simulink model "gm_sampleModel1485_3_sub"  (R2023a)
settings: Solver=VariableStepAuto  StartTime=0.0  StopTime=10.0  RelTol=1e-3
libraries: simulink x2, hdlsllib x1
settings Model: Creator=user1  LastModifiedBy=user1
settings OptimizationCC: BlockReduction=off  ConditionallyExecuteInputs=off
settings DebuggingCC: InheritedTsInSrcMsg=none

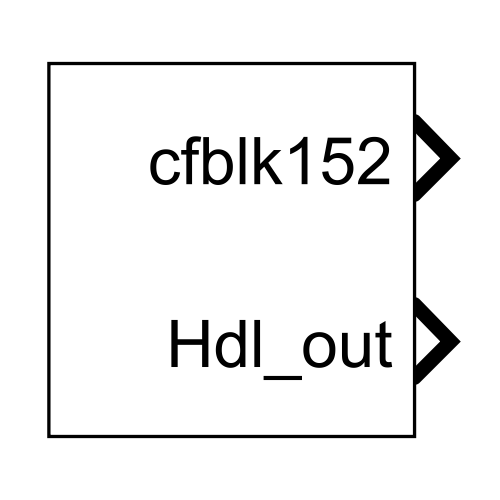
[thumbnail: Simulink's stored preview of the top-level diagram]
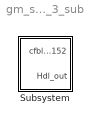
== system gm_sampleModel1485_3_sub ==
  Subsystem : Subsystem

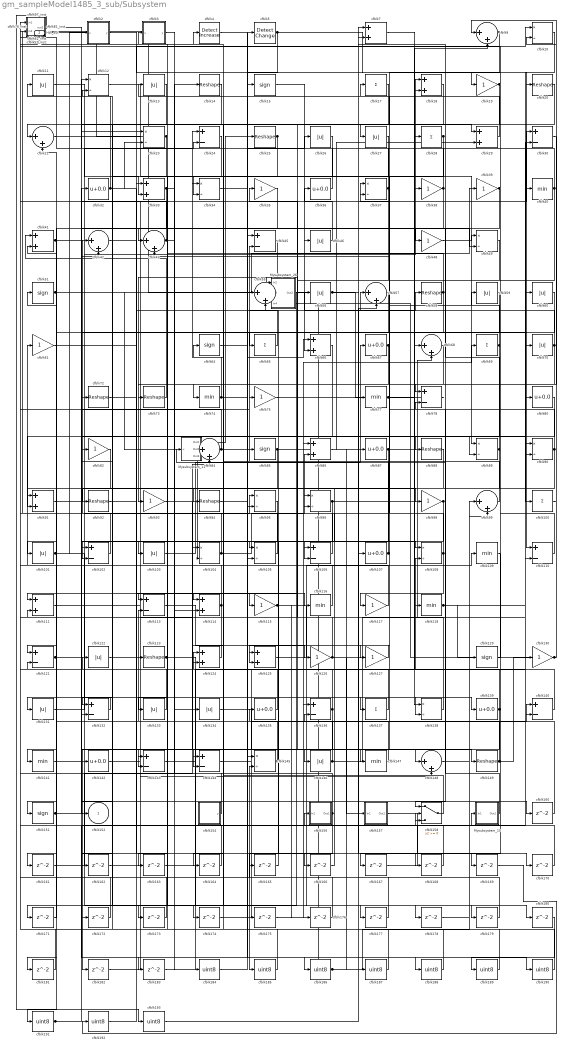
== system gm_sampleModel1485_3_sub/Subsystem ==
  Mysubsystem_10 : Subsystem
  Mysubsystem_11 : Subsystem
  Mysubsystem_26 : Subsystem
  cfblk{10,12,23,34,37,49,89..90,95..96,104..105,108,138,145} (15 alike) : Product  Inputs=*/  OutDataTypeStr=uint8  RndMeth=Zero  SaturateOnIntegerOverflow=on
  cfblk{17,28,65,69,100,137} (6 alike) : Sum  Inputs=+  OutDataTypeStr=uint8
  cfblk{11,13,26..27,46,56,59..60,70,101,103,122,131,133..134,146} (16 alike) : Abs  OutDataTypeStr=uint8  SaturateOnIntegerOverflow=off
  cfblk{24,30,45,78,102,106,110,113,121,132,136,140,143..144} (14 alike) : Sum  Inputs=+-  OutDataTypeStr=uint8
  cfblk{32,36,67,80,87,107,135,139,142} (9 alike) : Bias  Bias=0.0  SaturateOnIntegerOverflow=off
  cfblk{40,74,77,109,116,118,141,147} (8 alike) : MinMax  OutDataTypeStr=uint8
  cfblk{7,18,29,33,41,66,86,91,111,114,124..125} (12 alike) : Sum  OutDataTypeStr=uint8
  cfblk{19,35,38..39,48,61,75,82,93,98,115,117,126..127,130} (15 alike) : Gain  OutDataTypeStr=uint8
  cfblk{14,20,25,58,72..73,88,92,94,123,149} (11 alike) : Reshape
  cfblk{15,51,64,85,129,151} (6 alike) : Signum
  cfblk{9,21,42..43,55,57,68,84,99,148} (10 alike) : Sum  Inputs=|++  OutDataTypeStr=uint8
  cfblk150_inst : Subsystem
  cfblk154 : Subsystem  mask(Counter Free-Running){NumBits=double(16), tsamp=double(-1)}
      mask prompts: NumBits "Simulink:masks:NumberOfBits_MP"; tsamp "Simulink:masks:SampleTime_MP"
      mask help: Simulink:masks:CounterFreeRunning_MD
  cfblk156 : Subsystem
  cfblk157 : Subsystem
  cfblk158 : Switch  OutDataTypeStr=uint8  SaturateOnIntegerOverflow=off  InputSameDT=off
  cfblk{160..183} (24 alike) : Delay  SampleTime=1
  cfblk16_inst : Subsystem
  cfblk{184..193} (10 alike) : DataTypeConversion  OutDataTypeStr=uint8  SaturateOnIntegerOverflow=off  RndMeth=Floor
  cfblk2 : Subsystem  mask(Compare To Zero){relop=<=, OutDataTypeStr=uint8, ZeroCross=on}
      mask prompts: relop "Simulink:masks:Operator_MP"; OutDataTypeStr "Simulink:masks:OutputDataType_MP"; ZeroCross "Simulink:masks:EnableZerocrossingDetection_MP"
      mask help: Simulink:masks:CompareToZero_MD
      mask init:
      | OutDataTypeStr = 'uint8';
      | ZeroCross = 'on';
      | blkName = 'sampleModel1485_3_sub/Subsystem/cfblk2';
      | relop = '<=';
      | setValue = 'fixdt(0, 8)';
      mask TypeOptions relop: == | ~= | < | <= | >= | >
      mask TypeOptions OutDataTypeStr: Simulink:masks:uint8 | Simulink:masks:boolean
      mask Callback ZeroCross: sl('zeroCrossEnable', gcbh);
      mask Display: disp([relop,' 0'])
  cfblk22_inst : Subsystem
  cfblk3 : Subsystem  mask(Compare To Constant){relop=<=, const=double(3), OutDataTypeStr=uint8, ZeroCross=on}
      mask prompts: relop "Simulink:masks:Operator_MP"; const "Simulink:masks:ConstantValue_MP"; OutDataTypeStr "Simulink:masks:OutputDataType_MP"; ZeroCross "Simulink:masks:EnableZerocrossingDetection_MP"
      mask help: Simulink:masks:CompareToConstant_MD
      mask init:
      | OutDataTypeStr = 'uint8';
      | ZeroCross = 'on';
      | blkName = 'sampleModel1485_3_sub/Subsystem/cfblk3';
      | const = double(3);
      | const_str = '3.0';
      | const_val = double(3);
      | relop = '<=';
      | setValue = 'fixdt(0, 8)';
      | str = '<= 3';
      mask TypeOptions relop: == | ~= | < | <= | >= | >
      mask TypeOptions OutDataTypeStr: Simulink:masks:uint8 | Simulink:masks:boolean
      mask Callback ZeroCross: sl('zeroCrossEnable', gcbh);
      mask Display: disp(str)
  cfblk31_inst : Subsystem
  cfblk4 : simulink/Logic and Bit Operations/Detect Increase  vinit=0.0  OutDataTypeStr=uint8
      settings: LibrarySourceBlock=|
      | hdlsllib/Logic and Bit
      | Operations/Detect
      | Increase
  cfblk47_inst : Subsystem
  cfblk5 : simulink/Logic and Bit Operations/Detect Change  vinit=0  OutDataTypeStr=uint8
      settings: LibrarySourceBlock=|
      | hdlsllib/Logic and Bit
      | Operations/Detect
      | Change
  cfblk52_inst : Subsystem
  cfblk54_inst : Subsystem
  cfblk62_inst : Subsystem
  cfblk76_inst : Subsystem
  cfblk81_inst : Subsystem
  cfblk97_inst : Subsystem
  cfblk152 : Outport  OutDataTypeStr=uint8  SampleTime=1  VectorParamsAs1DForOutWhenUnconnected=off
  Hdl_out : Outport  Port=2  OutDataTypeStr=uint8  SampleTime=1
  wires:
  Mysubsystem_10/1(Out1) -> Mysubsystem_11/1(u)
  Mysubsystem_11/1(Out1) -> cfblk25/1
  Mysubsystem_11/2(Out2) -> cfblk29/2
  Mysubsystem_11/3(Out3) -> cfblk104/2
  Mysubsystem_26/1(Out2) -> cfblk171/1
  cfblk10/1 -> cfblk110/1
  cfblk100/1 -> cfblk9/1
  cfblk101/1 -> cfblk24/2, cfblk95/1, cfblk178/1, cfblk2/1(u)
  cfblk102/1 -> cfblk42/1
  cfblk103/1 -> cfblk67/1
  cfblk104/1 -> cfblk86/2, cfblk54_inst/2(in2)
  cfblk105/1 -> cfblk97_inst/1(in1)
  cfblk106/1 -> cfblk96/1
  cfblk107/1 -> cfblk45/2, cfblk150_inst/1(in1)
  cfblk108/1 -> cfblk45/1, cfblk117/1, cfblk17/1
  cfblk109/1 -> cfblk167/1
  cfblk11/1 -> cfblk33/2
  cfblk110/1 -> cfblk81_inst/2(in2)
  cfblk111/1 -> cfblk58/1
  cfblk113/1 -> cfblk125/2
  cfblk114/1 -> cfblk22_inst/1(in1), cfblk111/2
  cfblk115/1 -> cfblk177/1, cfblk176/1
  cfblk116/1 -> cfblk35/1
  cfblk117/1 -> cfblk61/1
  cfblk118/1 -> cfblk60/1, cfblk129/1
  cfblk12/1 -> cfblk89/1
  cfblk121/1 -> cfblk18/1, cfblk139/1, cfblk181/1
  cfblk122/1 -> cfblk5/1
  cfblk123/1 -> cfblk180/1, cfblk179/1
  cfblk124/1 -> cfblk16_inst/1(in1)
  cfblk125/1 -> cfblk109/1
  cfblk126/1 -> cfblk68/2, cfblk157/1(In1), Mysubsystem_26/1(In2)
  cfblk127/1 -> cfblk125/1
  cfblk129/1 -> cfblk59/1
  cfblk13/1 -> cfblk21/1
  cfblk130/1 -> cfblk10/2, Mysubsystem_26/3(In4)
  cfblk131/1 -> cfblk15/1
  cfblk132/1 -> cfblk131/1
  cfblk133/1 -> cfblk122/1
  cfblk134/1 -> cfblk149/1
  cfblk135/1 -> cfblk72/1
  cfblk136/1 -> cfblk85/1, cfblk182/1
  cfblk137/1 -> cfblk124/1
  cfblk138/1 -> cfblk97_inst/2(in2)
  cfblk139/1 -> cfblk142/1, cfblk108/2
  cfblk14/1 -> cfblk102/2
  cfblk140/1 -> cfblk47_inst/1(in1)
  cfblk141/1 -> cfblk75/1
  cfblk142/1 -> cfblk30/1
  cfblk143/1 -> cfblk18/2
  cfblk144/1 -> cfblk68/1
  cfblk145/1 -> cfblk51/1, cfblk135/1
  cfblk146/1 -> cfblk30/2, cfblk113/2
  cfblk147/1 -> cfblk136/2
  cfblk148/1 -> cfblk140/1
  cfblk149/1 -> cfblk78/2, cfblk130/1
  cfblk15/1 -> cfblk66/2
  cfblk150_inst/1(out1) -> cfblk193/1
  cfblk151/1 -> cfblk32/1, cfblk14/1
  cfblk154/1(y) -> cfblk121/2
  cfblk156/1(Out1) -> cfblk31_inst/1(in1), cfblk185/1
  cfblk157/1(Out1) -> cfblk170/1
  cfblk158/1 -> cfblk64/1
  cfblk16_inst/1(out1) -> cfblk42/2
  cfblk160/1 -> cfblk86/1
  cfblk161/1 -> cfblk104/1
  cfblk162/1 -> cfblk148/2
  cfblk163/1 -> cfblk158/2
  cfblk164/1 -> cfblk81_inst/1(in1)
  cfblk165/1 -> cfblk55/2
  cfblk166/1 -> cfblk96/2
  cfblk167/1 -> cfblk90/1
  cfblk168/1 -> cfblk33/1
  cfblk169/1 -> cfblk192/1
  cfblk17/1 -> cfblk102/1
  cfblk170/1 -> cfblk136/1
  cfblk171/1 -> cfblk21/2
  cfblk172/1 -> cfblk52_inst/1(in1)
  cfblk173/1 -> cfblk150_inst/2(in2)
  cfblk174/1 -> cfblk99/2
  cfblk175/1 -> cfblk158/3
  cfblk176/1 -> cfblk145/2
  cfblk177/1 -> cfblk12/2
  cfblk178/1 -> cfblk140/2
  cfblk179/1 -> cfblk41/2
  cfblk18/1 -> cfblk124/2
  cfblk180/1 -> cfblk189/1
  cfblk181/1 -> cfblk62_inst/2(in2)
  cfblk182/1 -> cfblk84/2
  cfblk183/1 -> cfblk110/2
  cfblk184/1 -> cfblk26/1
  cfblk185/1 -> cfblk3/1(u)
  cfblk186/1 -> cfblk99/1, cfblk87/1
  cfblk187/1 -> cfblk4/1
  cfblk188/1 -> cfblk82/1
  cfblk189/1 -> cfblk76_inst/1(in1)
  cfblk19/1 -> cfblk34/2, cfblk174/1
  cfblk190/1 -> cfblk76_inst/2(in2)
  cfblk191/1 -> cfblk156/1(In1), Mysubsystem_10/1(In1)
  cfblk192/1 -> cfblk57/1
  cfblk193/1 -> cfblk57/2
  cfblk2/1(y) -> cfblk20/1
  cfblk20/1 -> cfblk115/1
  cfblk21/1 -> cfblk118/1
  cfblk22_inst/1(out1) -> cfblk29/1
  cfblk23/1 -> Hdl_out/1, cfblk152/1
  cfblk24/1 -> cfblk172/1
  cfblk25/1 -> cfblk94/1, cfblk43/1
  cfblk26/1 -> cfblk46/1
  cfblk27/1 -> cfblk92/1
  cfblk28/1 -> cfblk173/1, cfblk127/1
  cfblk29/1 -> cfblk13/1
  cfblk3/1(y) -> cfblk184/1
  cfblk30/1 -> cfblk80/1
  cfblk31_inst/1(out1) -> cfblk65/1
  cfblk32/1 -> cfblk144/2, cfblk11/1, cfblk23/2
  cfblk33/1 -> cfblk91/2, cfblk134/1
  cfblk34/1 -> cfblk70/1
  cfblk35/1 -> cfblk161/1
  cfblk36/1 -> cfblk31_inst/2(in2)
  cfblk37/1 -> cfblk54_inst/1(in1), cfblk111/1
  cfblk38/1 -> cfblk28/1, cfblk74/1
  cfblk39/1 -> cfblk78/1, cfblk48/1
  cfblk4/1 -> cfblk186/1
  cfblk40/1 -> cfblk143/2, cfblk12/1
  cfblk41/1 -> cfblk151/1, cfblk37/1, cfblk160/1
  cfblk42/1 -> cfblk116/1
  cfblk43/1 -> cfblk22_inst/2(in2), cfblk114/2
  cfblk45/1 -> cfblk93/1
  cfblk46/1 -> cfblk36/1
  cfblk47_inst/1(out1) -> cfblk90/2
  cfblk48/1 -> cfblk49/1
  cfblk49/1 -> cfblk73/1
  cfblk5/1 -> cfblk175/1, cfblk100/1
  cfblk51/1 -> cfblk84/1, cfblk39/1
  cfblk52_inst/1(out1) -> cfblk190/1, cfblk23/1
  cfblk54_inst/1(out1) -> cfblk105/1, cfblk137/1
  cfblk55/1 -> cfblk47_inst/2(in2), cfblk187/1
  cfblk56/1 -> cfblk7/2, cfblk169/1
  cfblk57/1 -> cfblk191/1
  cfblk58/1 -> cfblk16_inst/2(in2), cfblk121/1
  cfblk59/1 -> cfblk148/1
  cfblk60/1 -> cfblk105/2
  cfblk61/1 -> cfblk123/1
  cfblk62_inst/1(out1) -> cfblk49/2
  cfblk64/1 -> cfblk145/1
  cfblk65/1 -> cfblk55/1
  cfblk66/1 -> cfblk91/1
  cfblk67/1 -> cfblk95/2, cfblk147/1
  cfblk68/1 -> cfblk164/1
  cfblk69/1 -> cfblk43/2, cfblk114/1
  cfblk7/1 -> cfblk38/1
  cfblk70/1 -> cfblk88/1, cfblk56/1
  cfblk72/1 -> cfblk10/1
  cfblk73/1 -> cfblk41/1
  cfblk74/1 -> cfblk24/1, cfblk126/1
  cfblk75/1 -> cfblk77/1
  cfblk76_inst/1(out1) -> cfblk188/1
  cfblk77/1 -> cfblk89/2, cfblk40/1
  cfblk78/1 -> Mysubsystem_26/2(In3)
  cfblk80/1 -> cfblk101/1
  cfblk81_inst/1(out1) -> cfblk103/1, cfblk183/1
  cfblk82/1 -> cfblk141/1
  cfblk84/1 -> cfblk62_inst/1(in1), cfblk138/2
  cfblk85/1 -> cfblk132/1, cfblk69/1
  cfblk86/1 -> cfblk107/1
  cfblk87/1 -> cfblk9/2, cfblk106/2
  cfblk88/1 -> cfblk113/1
  cfblk89/1 -> cfblk7/1, cfblk158/1, cfblk132/2
  cfblk9/1 -> cfblk27/1, cfblk19/1
  cfblk90/1 -> cfblk106/1, cfblk37/2
  cfblk91/1 -> cfblk34/1
  cfblk92/1 -> cfblk168/1
  cfblk93/1 -> cfblk146/1
  cfblk94/1 -> cfblk66/1
  cfblk95/1 -> cfblk133/1
  cfblk96/1 -> cfblk162/1, cfblk138/1
  cfblk97_inst/1(out1) -> cfblk143/1, cfblk98/1, cfblk166/1, cfblk108/1
  cfblk98/1 -> cfblk144/1, cfblk165/1, cfblk163/1
  cfblk99/1 -> cfblk52_inst/2(in2)

== system gm_sampleModel1485_3_sub/Subsystem/Mysubsystem_10 ==
  In1 : Inport  OutDataTypeStr=uint8  PortDimensions=1  SampleTime=1
  cfblk159 : Delay  SampleTime=1
  Out1 : Outport  SampleTime=1
  wires:
  In1/1 -> cfblk159/1
  cfblk159/1 -> Out1/1

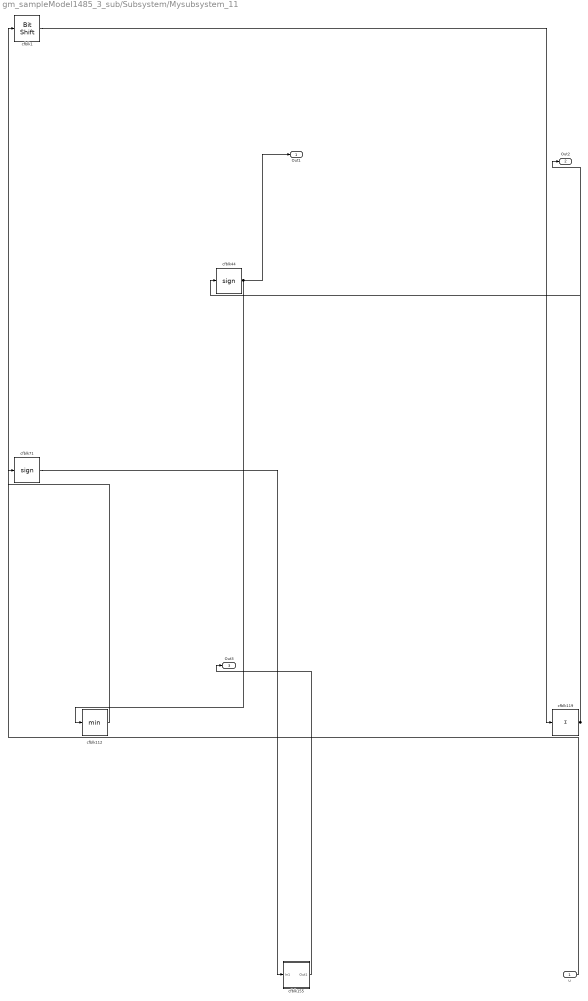
== system gm_sampleModel1485_3_sub/Subsystem/Mysubsystem_11 ==
  u : Inport  OutDataTypeStr=uint8  PortDimensions=1  SampleTime=1
  cfblk1 : hdlsllib/Logic and Bit Operations/Bit Shift  mode=Shift Left Logical  N=0
  cfblk112 : MinMax
  cfblk119 : Sum  Inputs=+
  cfblk155 : Subsystem
  cfblk44 : Signum
  cfblk71 : Signum
  Out1 : Outport  SampleTime=1
  Out2 : Outport  Port=2  SampleTime=1
  Out3 : Outport  Port=3  SampleTime=1
  wires:
  u/1 -> cfblk1/1
  cfblk1/1 -> cfblk119/1
  cfblk112/1 -> cfblk71/1
  cfblk119/1 -> cfblk44/1, Out2/1
  cfblk155/1(Out1) -> Out3/1
  cfblk44/1 -> Out1/1, cfblk112/1
  cfblk71/1 -> cfblk155/1(In1)

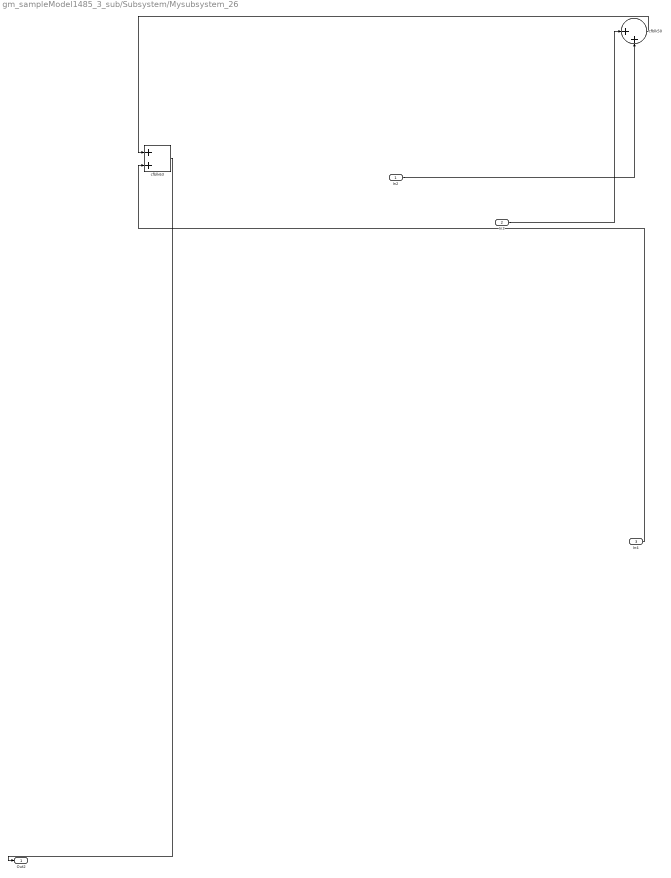
== system gm_sampleModel1485_3_sub/Subsystem/Mysubsystem_26 ==
  In2 : Inport  OutDataTypeStr=uint8  PortDimensions=1  SampleTime=1
  In3 : Inport  Port=2  OutDataTypeStr=uint8  PortDimensions=1  SampleTime=1
  In4 : Inport  Port=3  OutDataTypeStr=uint8  PortDimensions=1  SampleTime=1
  cfblk50 : Sum  Inputs=|++
  cfblk63 : Sum
  Out2 : Outport  SampleTime=1
  wires:
  In2/1 -> cfblk50/2
  In3/1 -> cfblk50/1
  In4/1 -> cfblk63/2
  cfblk50/1 -> cfblk63/1
  cfblk63/1 -> Out2/1

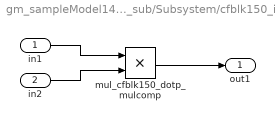
== system gm_sampleModel1485_3_sub/Subsystem/cfblk150_inst ==
  in1 : Inport  OutDataTypeStr=uint8  SampleTime=1
  in2 : Inport  Port=2  OutDataTypeStr=uint8  SampleTime=1
  mul_cfblk150_dotp_mulcomp : Product  Inputs=**  OutDataTypeStr=uint8  SampleTime=1
  out1 : Outport  OutDataTypeStr=uint8  SampleTime=1
  wires:
  in1/1 -> mul_cfblk150_dotp_mulcomp/1
  in2/1 -> mul_cfblk150_dotp_mulcomp/2
  mul_cfblk150_dotp_mulcomp/1 -> out1/1

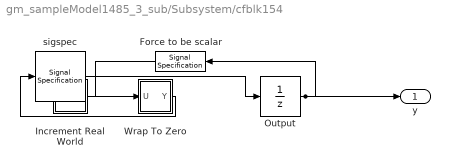
== system gm_sampleModel1485_3_sub/Subsystem/cfblk154 ==
  Force to be scalar : SignalSpecification  DisableCoverage=on  Dimensions=1
  Increment Real World : Subsystem  mask(Real World Value Increment){}
      mask help: Simulink:masks:RealWorldValueIncrement_MD
      mask Display: disp('V++')
  Output : UnitDelay  InitialCondition=0.0  SampleTime=tsamp  HasFrameUpgradeWarning=on
  Wrap To Zero : Subsystem  mask(Wrap To Zero){Threshold=double(65535)}
      mask prompts: Threshold "Simulink:masks:Threshold_MP"
      mask help: Simulink:masks:WrapToZero_MD
  sigspec : SignalSpecification  OutDataTypeStr=uint16  Dimensions=1
  y : Outport  SampleTime=1
  wires:
  Force to be scalar/1 -> Increment Real World/1(u)
  Increment Real World/1(y) -> Wrap To Zero/1(U)
  Output/1 -> Force to be scalar/1, y/1
  Wrap To Zero/1(Y) -> sigspec/1
  sigspec/1 -> Output/1

== system gm_sampleModel1485_3_sub/Subsystem/cfblk156 ==
  In1 : Inport  OutDataTypeStr=uint8  PortDimensions=1  SampleTime=1
  Out1 : Outport  SampleTime=1
  wires:
  In1/1 -> Out1/1

== system gm_sampleModel1485_3_sub/Subsystem/cfblk157 ==
  In1 : Inport  OutDataTypeStr=uint8  PortDimensions=1  SampleTime=1
  Out1 : Outport  SampleTime=1
  wires:
  In1/1 -> Out1/1

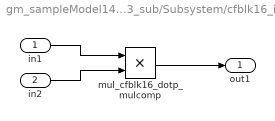
== system gm_sampleModel1485_3_sub/Subsystem/cfblk16_inst ==
  in1 : Inport  OutDataTypeStr=uint8  SampleTime=1
  in2 : Inport  Port=2  OutDataTypeStr=uint8  SampleTime=1
  mul_cfblk16_dotp_mulcomp : Product  Inputs=**  OutDataTypeStr=uint8  SampleTime=1
  out1 : Outport  OutDataTypeStr=uint8  SampleTime=1
  wires:
  in1/1 -> mul_cfblk16_dotp_mulcomp/1
  in2/1 -> mul_cfblk16_dotp_mulcomp/2
  mul_cfblk16_dotp_mulcomp/1 -> out1/1

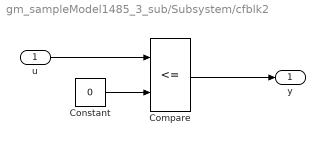
== system gm_sampleModel1485_3_sub/Subsystem/cfblk2 ==
  u : Inport  OutDataTypeStr=uint8  SampleTime=1
  Compare : RelationalOperator  Operator=<=  OutDataTypeStr=fixdt(0, 8)
  Constant : Constant  DisableCoverage=on  Value=0  OutDataTypeStr=Inherit: Inherit via back propagation  SampleTime=-1  PreserveConstantTs=on
  y : Outport  SampleTime=1
  wires:
  u/1 -> Compare/1
  Compare/1 -> y/1
  Constant/1 -> Compare/2

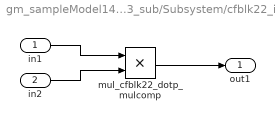
== system gm_sampleModel1485_3_sub/Subsystem/cfblk22_inst ==
  in1 : Inport  OutDataTypeStr=uint8  SampleTime=1
  in2 : Inport  Port=2  OutDataTypeStr=uint8  SampleTime=1
  mul_cfblk22_dotp_mulcomp : Product  Inputs=**  OutDataTypeStr=uint8  SampleTime=1
  out1 : Outport  OutDataTypeStr=uint8  SampleTime=1
  wires:
  in1/1 -> mul_cfblk22_dotp_mulcomp/1
  in2/1 -> mul_cfblk22_dotp_mulcomp/2
  mul_cfblk22_dotp_mulcomp/1 -> out1/1

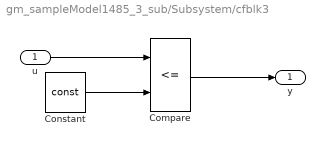
== system gm_sampleModel1485_3_sub/Subsystem/cfblk3 ==
  u : Inport  OutDataTypeStr=uint8  SampleTime=1
  Compare : RelationalOperator  Operator=<=  OutDataTypeStr=fixdt(0, 8)
  Constant : Constant  DisableCoverage=on  Value=const  OutDataTypeStr=Inherit: Inherit via back propagation  SampleTime=-1
  y : Outport  SampleTime=1
  wires:
  u/1 -> Compare/1
  Compare/1 -> y/1
  Constant/1 -> Compare/2

== system gm_sampleModel1485_3_sub/Subsystem/cfblk31_inst ==
  in1 : Inport  OutDataTypeStr=uint8  SampleTime=1
  in2 : Inport  Port=2  OutDataTypeStr=uint8  SampleTime=1
  mul_cfblk31_dotp_mulcomp : Product  Inputs=**  OutDataTypeStr=uint8  SampleTime=1
  out1 : Outport  OutDataTypeStr=uint8  SampleTime=1
  wires:
  in1/1 -> mul_cfblk31_dotp_mulcomp/1
  in2/1 -> mul_cfblk31_dotp_mulcomp/2
  mul_cfblk31_dotp_mulcomp/1 -> out1/1

== system gm_sampleModel1485_3_sub/Subsystem/cfblk47_inst ==
  in1 : Inport  OutDataTypeStr=uint8  SampleTime=1
  in2 : Inport  Port=2  OutDataTypeStr=uint8  SampleTime=1
  mul_cfblk47_dotp_mulcomp : Product  Inputs=**  OutDataTypeStr=uint8  SampleTime=1
  out1 : Outport  OutDataTypeStr=uint8  SampleTime=1
  wires:
  in1/1 -> mul_cfblk47_dotp_mulcomp/1
  in2/1 -> mul_cfblk47_dotp_mulcomp/2
  mul_cfblk47_dotp_mulcomp/1 -> out1/1

== system gm_sampleModel1485_3_sub/Subsystem/cfblk52_inst ==
  in1 : Inport  OutDataTypeStr=uint8  SampleTime=1
  in2 : Inport  Port=2  OutDataTypeStr=uint8  SampleTime=1
  mul_cfblk52_dotp_mulcomp : Product  Inputs=**  OutDataTypeStr=uint8  SampleTime=1
  out1 : Outport  OutDataTypeStr=uint8  SampleTime=1
  wires:
  in1/1 -> mul_cfblk52_dotp_mulcomp/1
  in2/1 -> mul_cfblk52_dotp_mulcomp/2
  mul_cfblk52_dotp_mulcomp/1 -> out1/1

== system gm_sampleModel1485_3_sub/Subsystem/cfblk54_inst ==
  in1 : Inport  OutDataTypeStr=uint8  SampleTime=1
  in2 : Inport  Port=2  OutDataTypeStr=uint8  SampleTime=1
  mul_cfblk54_dotp_mulcomp : Product  Inputs=**  OutDataTypeStr=uint8  SampleTime=1
  out1 : Outport  OutDataTypeStr=uint8  SampleTime=1
  wires:
  in1/1 -> mul_cfblk54_dotp_mulcomp/1
  in2/1 -> mul_cfblk54_dotp_mulcomp/2
  mul_cfblk54_dotp_mulcomp/1 -> out1/1

== system gm_sampleModel1485_3_sub/Subsystem/cfblk62_inst ==
  in1 : Inport  OutDataTypeStr=uint8  SampleTime=1
  in2 : Inport  Port=2  OutDataTypeStr=uint8  SampleTime=1
  mul_cfblk62_dotp_mulcomp : Product  Inputs=**  OutDataTypeStr=uint8  SampleTime=1
  out1 : Outport  OutDataTypeStr=uint8  SampleTime=1
  wires:
  in1/1 -> mul_cfblk62_dotp_mulcomp/1
  in2/1 -> mul_cfblk62_dotp_mulcomp/2
  mul_cfblk62_dotp_mulcomp/1 -> out1/1

== system gm_sampleModel1485_3_sub/Subsystem/cfblk76_inst ==
  in1 : Inport  OutDataTypeStr=uint8  SampleTime=1
  in2 : Inport  Port=2  OutDataTypeStr=uint8  SampleTime=1
  mul_cfblk76_dotp_mulcomp : Product  Inputs=**  OutDataTypeStr=uint8  SampleTime=1
  out1 : Outport  OutDataTypeStr=uint8  SampleTime=1
  wires:
  in1/1 -> mul_cfblk76_dotp_mulcomp/1
  in2/1 -> mul_cfblk76_dotp_mulcomp/2
  mul_cfblk76_dotp_mulcomp/1 -> out1/1

== system gm_sampleModel1485_3_sub/Subsystem/cfblk81_inst ==
  in1 : Inport  OutDataTypeStr=uint8  SampleTime=1
  in2 : Inport  Port=2  OutDataTypeStr=uint8  SampleTime=1
  mul_cfblk81_dotp_mulcomp : Product  Inputs=**  OutDataTypeStr=uint8  SampleTime=1
  out1 : Outport  OutDataTypeStr=uint8  SampleTime=1
  wires:
  in1/1 -> mul_cfblk81_dotp_mulcomp/1
  in2/1 -> mul_cfblk81_dotp_mulcomp/2
  mul_cfblk81_dotp_mulcomp/1 -> out1/1

== system gm_sampleModel1485_3_sub/Subsystem/cfblk97_inst ==
  in1 : Inport  OutDataTypeStr=uint8  SampleTime=1
  in2 : Inport  Port=2  OutDataTypeStr=uint8  SampleTime=1
  mul_cfblk97_dotp_mulcomp : Product  Inputs=**  OutDataTypeStr=uint8  SampleTime=1
  out1 : Outport  OutDataTypeStr=uint8  SampleTime=1
  wires:
  in1/1 -> mul_cfblk97_dotp_mulcomp/1
  in2/1 -> mul_cfblk97_dotp_mulcomp/2
  mul_cfblk97_dotp_mulcomp/1 -> out1/1

== system gm_sampleModel1485_3_sub/Subsystem/Mysubsystem_11/cfblk155 ==
  In1 : Inport  OutDataTypeStr=uint8  PortDimensions=1  SampleTime=1
  Out1 : Outport  SampleTime=1
  wires:
  In1/1 -> Out1/1

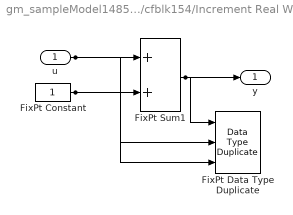
== system gm_sampleModel1485_3_sub/Subsystem/cfblk154/Increment Real World ==
  u : Inport  OutDataTypeStr=uint16  SampleTime=1
  FixPt Constant : Constant  DisableCoverage=on  OutDataTypeStr=Inherit: Inherit via back propagation  SampleTime=-1
  FixPt Data Type Duplicate : DataTypeDuplicate  DisableCoverage=on  NumInputPorts=3
  FixPt Sum1 : Sum  InputSameDT=on  OutDataTypeStr=Inherit: Inherit via back propagation  LockScale=on
  y : Outport  SampleTime=1
  wires:
  u/1 -> FixPt Sum1/1, FixPt Data Type Duplicate/2
  FixPt Constant/1 -> FixPt Sum1/2, FixPt Data Type Duplicate/3
  FixPt Sum1/1 -> FixPt Data Type Duplicate/1, y/1

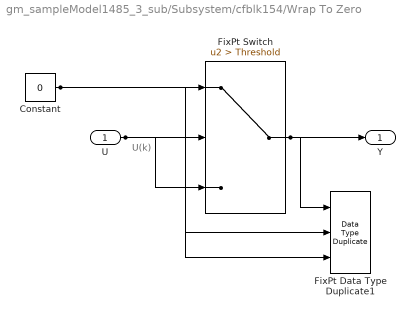
== system gm_sampleModel1485_3_sub/Subsystem/cfblk154/Wrap To Zero ==
  note: U(k)
  U : Inport  OutDataTypeStr=uint16  SampleTime=1
  Constant : Constant  DisableCoverage=on  Value=0  OutDataTypeStr=Inherit: Inherit via back propagation  SampleTime=-1
  FixPt Data Type Duplicate1 : DataTypeDuplicate  DisableCoverage=on  NumInputPorts=3
  FixPt Switch : Switch  Criteria=u2 > Threshold  Threshold=Threshold  OutDataTypeStr=Inherit: Inherit via back propagation  ZeroCross=off  SaturateOnIntegerOverflow=off  InputSameDT=off
  Y : Outport  SampleTime=1
  wires:
  U/1 -> FixPt Switch/3, FixPt Switch/2, FixPt Data Type Duplicate1/2
  Constant/1 -> FixPt Switch/1, FixPt Data Type Duplicate1/3
  FixPt Switch/1 -> FixPt Data Type Duplicate1/1, Y/1
